simulink model "model_fully_coupled"  (R2021a)
settings: Solver=ode4  StartTime=0.0  StopTime=4  FixedStep=1e-2  RelTol=1e-3
values from neighbouring files (symbols this model uses):
  C_1 = [0.7887 -0.2113 -0.5774; -0.2113 0.7887 -0.5774; 0.5774 0.5774 0.5774]    [parameter.m]
  C_2 = [-0.2113 -0.5774 0.7887; 0.7887 -0.5774 -0.2113; 0.5774 0.5774 0.5774]    [parameter.m]
  C_3 = [-0.5774 0.7887 -0.2113; -0.5774 -0.2113 0.7887; 0.5774 0.5774 0.5774]    [parameter.m]
  d_1 = d    (= 4e-07)    [parameter.m]
  d_2 = d    (= 4e-07)    [parameter.m]
  d_3 = d    (= 4e-07)    [parameter.m]
  F = [0;0;0]    [parameter.m]
  g_s_1 = C_1(1:3,1)    [parameter.m]
  g_s_2 = C_2(1:3,1)    [parameter.m]
  g_s_3 = C_3(1:3,1)    [parameter.m]
  I = [1 0 0;0 1 0;0 0 1]    [parameter.m]
  I_hub_Bc = [550 0.1045 -0.0840; 0.1045 650 0.0001; -0.0840 0.0001 650]    [parameter.m]
  I_rw1_Wc1 = [1.5915E-4 0 1.54E-10; 0 0.8594E-4 0; 1.54E-10 0 0.8594E-4]    [parameter.m]
  I_rw1_Wc1_ = [0 -J_13_1 J_12_1; -J_13_1 (-2*J_23_1) (J_22_1-J_33_1); J_12_1 (J_22_1-J_33_1) (-2*J_23_1)]    [parameter.m]
  I_rw2_Wc2 = [1.5915E-4 0 1.54E-10; 0 0.8594E-4 0; 1.54E-10 0 0.8594E-4]    [parameter.m]
  I_rw2_Wc2_ = [0 -J_13_2 J_12_2; -J_13_2 (-2*J_23_2) (J_22_2-J_33_2); J_12_2 (J_22_2-J_33_2) (-2*J_23_2)]    [parameter.m]
  I_rw3_Wc3 = [1.5915E-4 0 1.54E-10; 0 0.8594E-4 0; 1.54E-10 0 0.8594E-4]    [parameter.m]
  I_rw3_Wc3_ = [0 -J_13_3 J_12_3; -J_13_3 (-2*J_23_3) (J_22_3-J_33_3); J_12_3 (J_22_3-J_33_3) (-2*J_23_3)]    [parameter.m]
  J_11_1 = I_rw1_Wc1(1,1)    [parameter.m]
  J_11_2 = I_rw2_Wc2(1,1)    [parameter.m]
  J_11_3 = I_rw3_Wc3(1,1)    [parameter.m]
  J_12_1 = I_rw1_Wc1(1,2)    [parameter.m]
  J_12_2 = I_rw2_Wc2(1,2)    [parameter.m]
  J_12_3 = I_rw3_Wc3(1,2)    [parameter.m]
  J_13_1 = I_rw1_Wc1(1,3)    [parameter.m]
  J_13_2 = I_rw2_Wc2(1,3)    [parameter.m]
  J_13_3 = I_rw3_Wc3(1,3)    [parameter.m]
  J_22_1 = I_rw1_Wc1(2,2)    [parameter.m]
  J_22_2 = I_rw2_Wc2(2,2)    [parameter.m]
  J_22_3 = I_rw3_Wc3(2,2)    [parameter.m]
  J_23_1 = I_rw1_Wc1(2,3)    [parameter.m]
  J_23_2 = I_rw2_Wc2(2,3)    [parameter.m]
  J_23_3 = I_rw3_Wc3(2,3)    [parameter.m]
  J_33_1 = I_rw1_Wc1(3,3)    [parameter.m]
  J_33_2 = I_rw2_Wc2(3,3)    [parameter.m]
  J_33_3 = I_rw3_Wc3(3,3)    [parameter.m]
  m_hub = 644    [parameter.m]
  m_rw_1 = m_rw(1)    [parameter.m]
  m_rw_2 = m_rw(2)    [parameter.m]
  m_rw_3 = m_rw(3)    [parameter.m]
  m_sc = 680    [parameter.m]
  OMEGA_1 = OMEGA(1)    [parameter.m]
  OMEGA_2 = OMEGA(2)    [parameter.m]
  OMEGA_3 = OMEGA(3)    [parameter.m]
  omega_BN = [omega ; omega; omega]    [parameter.m]
  r_Bc_B = [1e-2; -2e-2; 10e-2]    [parameter.m]
  r_BN = [0;0;0]    [parameter.m]
  r_W1_B = [0.6309; -0.1691; 0.4619]    [parameter.m]
  r_W2_B = [-0.1691; 0.6309; 0.4619]    [parameter.m]
  r_W3_B = [-0.4619; -0.4619; 0.4619]    [parameter.m]
  sigma_BN = [sigma; sigma; sigma]    [parameter.m]
  u_s_1 = u_s(1)    [parameter.m]
  u_s_2 = u_s(2)    [parameter.m]
  u_s_3 = u_s(3)    [parameter.m]
  w_2_1 = C_1(1:3,2)    [parameter.m]
  w_2_2 = C_2(1:3,2)    [parameter.m]
  w_2_3 = C_3(1:3,2)    [parameter.m]
  w_3_1 = C_1(1:3,3)    [parameter.m]
  w_3_2 = C_2(1:3,3)    [parameter.m]
  w_3_3 = C_3(1:3,3)    [parameter.m]
undefined symbols (not defined in the file or in its folder): deg, magnitude, rad, s
libraries: aerolibconvert2 x4, sharedutil x1, aerolibutil x1
(part 2 of 3)

== system model_fully_coupled/omega_dot_BN/6/1 ==
  I_rw1_Wc1 : Inport
  g_s_1 : Inport  Port=2
  m_rw_1 : Inport  Port=3
  OMEGA_1 : Inport  Port=4
  Add : Sum
  Matrix Multiply4 : Product  Multiplication=Matrix(*)
  Matrix Multiply5 : Product  Multiplication=Matrix(*)
  Product1 : Product
  Product2 : Product
  Out1 : Outport
  wires:
  Matrix Multiply4/1 -> Add/1
  Matrix Multiply5/1 -> Product2/2
  Product1/1 -> Matrix Multiply4/2
  Product2/1 -> Add/2
  g_s_1/1 -> Product1/2
  m_rw_1/1 -> Product2/1
  I_rw1_Wc1/1 -> Matrix Multiply4/1
  OMEGA_1/1 -> Product1/1
  Add/1 -> Out1/1
  [r_Wc1_B_skew] -> Matrix Multiply5/1
  [r_prime_Wc1_B] -> Matrix Multiply5/2

== system model_fully_coupled/omega_dot_BN/6/2 ==
  I_rw2_Wc2 : Inport
  g_s_2 : Inport  Port=2
  m_rw_2 : Inport  Port=3
  OMEGA_2 : Inport  Port=4
  Add1 : Sum
  Matrix Multiply1 : Product  Multiplication=Matrix(*)
  Matrix Multiply2 : Product  Multiplication=Matrix(*)
  Product3 : Product
  Product4 : Product
  Out2 : Outport
  wires:
  Matrix Multiply1/1 -> Add1/1
  Matrix Multiply2/1 -> Product4/2
  Product3/1 -> Matrix Multiply1/2
  I_rw2_Wc2/1 -> Matrix Multiply1/1
  m_rw_2/1 -> Product4/1
  Product4/1 -> Add1/2
  g_s_2/1 -> Product3/2
  Add1/1 -> Out2/1
  OMEGA_2/1 -> Product3/1
  [r_Wc2_B_skew] -> Matrix Multiply2/1
  [r_prime_Wc2_B] -> Matrix Multiply2/2

== system model_fully_coupled/omega_dot_BN/6/3 ==
  I_rw3_Wc3 : Inport
  g_s_3 : Inport  Port=2
  m_rw_3 : Inport  Port=3
  OMEGA_3 : Inport  Port=4
  Add2 : Sum
  Matrix Multiply3 : Product  Multiplication=Matrix(*)
  Matrix Multiply6 : Product  Multiplication=Matrix(*)
  Product5 : Product
  Product6 : Product
  Out3 : Outport
  wires:
  OMEGA_3/1 -> Product5/1
  Matrix Multiply3/1 -> Add2/1
  Matrix Multiply6/1 -> Product6/2
  m_rw_3/1 -> Product6/1
  Product6/1 -> Add2/2
  [r_Wc3_B_skew] -> Matrix Multiply6/1
  g_s_3/1 -> Product5/2
  I_rw3_Wc3/1 -> Matrix Multiply3/1
  Add2/1 -> Out3/1
  Product5/1 -> Matrix Multiply3/2
  [r_prime_Wc3_B] -> Matrix Multiply6/2

== system model_fully_coupled/omega_dot_BN/6/I_rwi_Wci ==
  Out1 : Outport
  Out2 : Outport  Port=2
  Out3 : Outport  Port=3
  wires:
  [I_rw1_Wc1] -> Out1/1
  [I_rw3_Wc3] -> Out3/1
  [I_rw2_Wc2] -> Out2/1

== system model_fully_coupled/omega_dot_BN/6/g_s_i ==
  g_s_1 : Constant  Value=g_s_1
  g_s_2 : Constant  Value=g_s_2
  g_s_3 : Constant  Value=g_s_3
  Out1 : Outport
  Out2 : Outport  Port=2
  Out3 : Outport  Port=3
  wires:
  g_s_3/1 -> Out3/1
  g_s_1/1 -> Out1/1
  g_s_2/1 -> Out2/1

== system model_fully_coupled/omega_dot_BN/6/m_rw_i ==
  m_rw_1 : Constant  Value=m_rw_1
  m_rw_2 : Constant  Value=m_rw_2
  m_rw_3 : Constant  Value=m_rw_3
  Out1 : Outport
  Out2 : Outport  Port=2
  Out3 : Outport  Port=3
  wires:
  m_rw_1/1 -> Out1/1
  m_rw_3/1 -> Out3/1
  m_rw_2/1 -> Out2/1

== system model_fully_coupled/omega_dot_BN/7 /m_rw_i ==
  m_rw_1 : Constant  Value=m_rw_1
  m_rw_2 : Constant  Value=m_rw_2
  m_rw_3 : Constant  Value=m_rw_3
  Out1 : Outport
  Out2 : Outport  Port=2
  Out3 : Outport  Port=3
  wires:
  m_rw_1/1 -> Out1/1
  m_rw_3/1 -> Out3/1
  m_rw_2/1 -> Out2/1

== system model_fully_coupled/r_double_dot_BN/c_double_dot/2 ==
  omega_BN : Inport
  c' : Inport  Port=2
  Gain : Gain  Gain=2
  Matrix Multiply1 : Product  Multiplication=Matrix(*)
  Subsystem1 : Subsystem
  1 : Outport
  tag scope: omega_BN_skew=global
  wires:
  omega_BN/1 -> Subsystem1/1(" ")
  Subsystem1/1("skew ") -> [omega_BN_skew], Matrix Multiply1/1
  c'/1 -> Matrix Multiply1/2
  Matrix Multiply1/1 -> Gain/1
  Gain/1 -> 1/1

== system model_fully_coupled/r_double_dot_BN/c_double_dot/3 ==
  omega_dot_BN : Inport
  c : Inport  Port=2
  Matrix Multiply1 : Product  Multiplication=Matrix(*)
  Subsystem1 : Subsystem
  1 : Outport
  wires:
  omega_dot_BN/1 -> Subsystem1/1(" ")
  Matrix Multiply1/1 -> 1/1
  Subsystem1/1("skew ") -> Matrix Multiply1/1
  c/1 -> Matrix Multiply1/2

== system model_fully_coupled/r_double_dot_BN/c_double_dot/4 ==
  c : Inport
  Matrix Multiply : Product  Multiplication=Matrix(*)
  Matrix Multiply1 : Product  Multiplication=Matrix(*)
  1 : Outport
  wires:
  Matrix Multiply/1 -> 1/1
  Matrix Multiply1/1 -> Matrix Multiply/2
  c/1 -> Matrix Multiply1/2
  [omega_BN_skew] -> Matrix Multiply1/1, Matrix Multiply/1

== system model_fully_coupled/r_double_dot_BN/c_double_dot/Subsystem1 ==
  In1 : Inport
  Demux : Demux  Outputs=3
  skew : MATLAB Function  TreatAsAtomicUnit=on
  "skew " : Outport
  wires:
  In1/1 -> Demux/1
  Demux/3 -> skew/3(a_3)
  Demux/2 -> skew/2(a_2)
  Demux/1 -> skew/1(a_1)
  skew/1(skew) -> "skew "/1

== system model_fully_coupled/r_double_dot_BN/c_double_dot/c ==
  Add : Sum  Inputs=+++
  Add1 : Sum
  Gain : Gain  Gain=1/m_sc
  Product{,1..3} (4 alike) : Product
  m_hub : Constant  Value=m_hub
  m_rw_i : Subsystem
  c : Outport
  wires:
  Add/1 -> Add1/2
  m_hub/1 -> Product/1
  Product1/1 -> Add/1
  [r_Bc_B] -> Product/2
  Product3/1 -> Add/3
  Product2/1 -> Add/2
  Product/1 -> Add1/1
  Add1/1 -> Gain/1
  Gain/1 -> c/1
  m_rw_i/1(Out1) -> Product1/1
  [r_Wc1_B] -> Product1/2
  m_rw_i/2(Out2) -> Product2/1
  [r_Wc2_B] -> Product2/2
  m_rw_i/3(Out3) -> Product3/1
  [r_Wc3_B] -> Product3/2

== system model_fully_coupled/r_double_dot_BN/c_double_dot/c" ==
  Add : Sum  Inputs=+++
  Gain : Gain  Gain=1/m_sc
  Product1 : Product
  Product2 : Product
  Product3 : Product
  m_rw_i : Subsystem
  "c\"" : Outport
  wires:
  Gain/1 -> "c\""/1
  Product1/1 -> Add/2
  Add/1 -> Gain/1
  Product2/1 -> Add/1
  Product3/1 -> Add/3
  [r_dprime_Wc1_B] -> Product2/2
  m_rw_i/1(Out1) -> Product2/1
  [r_dprime_Wc2_B] -> Product1/2
  m_rw_i/2(Out2) -> Product1/1
  m_rw_i/3(Out3) -> Product3/1
  [r_dprime_Wc3_B] -> Product3/2

== system model_fully_coupled/r_double_dot_BN/c_double_dot/c' ==
  Add : Sum  Inputs=+++
  Gain : Gain  Gain=1/m_sc
  Product1 : Product
  Product2 : Product
  Product3 : Product
  m_rw_i : Subsystem
  c' : Outport
  wires:
  Gain/1 -> c'/1
  Product1/1 -> Add/2
  Add/1 -> Gain/1
  Product2/1 -> Add/1
  Product3/1 -> Add/3
  [r_prime_Wc1_B] -> Product2/2
  m_rw_i/1(Out1) -> Product2/1
  [r_prime_Wc2_B] -> Product1/2
  m_rw_i/2(Out2) -> Product1/1
  m_rw_i/3(Out3) -> Product3/1
  [r_prime_Wc3_B] -> Product3/2

== system model_fully_coupled/r_double_dot_BN/c_double_dot/r_dprime_Wci_B ==
  OMEGA_1 : Inport
  OMEGA_2 : Inport  Port=2
  OMEGA_3 : Inport  Port=3
  w_2_1 : Inport  Port=4
  w_2_2 : Inport  Port=5
  w_2_3 : Inport  Port=6
  r_Wci_B' : Subsystem
  wires:
  w_2_3/1 -> r_Wci_B'/6(w_2_3)
  w_2_2/1 -> r_Wci_B'/5(w_2_2)
  w_2_1/1 -> r_Wci_B'/4(w_2_1)
  OMEGA_1/1 -> r_Wci_B'/1(OMEGA_1)
  OMEGA_2/1 -> r_Wci_B'/2(OMEGA_2)
  OMEGA_3/1 -> r_Wci_B'/3(OMEGA_3)

== system model_fully_coupled/r_double_dot_BN/c_double_dot/w_2_i dan w_3_i ==
  OMEGA_1 : Inport
  OMEGA_2 : Inport  Port=2
  OMEGA_3 : Inport  Port=3
  Subsystem : Subsystem
  Subsystem1 : Subsystem
  wires:
  OMEGA_1/1 -> Subsystem/1(OMEGA_1), Subsystem1/1(OMEGA_1)
  OMEGA_3/1 -> Subsystem/3(OMEGA_3), Subsystem1/3(OMEGA_3)
  OMEGA_2/1 -> Subsystem/2(OMEGA_2), Subsystem1/2(OMEGA_2)

== system model_fully_coupled/H_sc_B/2/H_rw1_B/Subsystem ==
  OMEGA_1 : Inport
  d_1 : Inport  Port=2
  w_3_1 : Inport  Port=3
  Add : Sum
  Matrix Multiply : Product  Multiplication=Matrix(*)
  Product1 : Product
  Product2 : Product
  Out1 : Outport
  wires:
  d_1/1 -> Product1/1
  Product1/1 -> Product2/2
  w_3_1/1 -> Product1/2
  [omega_BN_skew] -> Matrix Multiply/1
  OMEGA_1/1 -> Product2/1
  Product2/1 -> Add/1
  Matrix Multiply/1 -> Add/2
  Add/1 -> Out1/1
  [r_Wc1_B] -> Matrix Multiply/2

== system model_fully_coupled/H_sc_B/2/H_rw2_B/Subsystem ==
  OMEGA_2 : Inport
  d_2 : Inport  Port=2
  w_3_2 : Inport  Port=3
  Add : Sum
  Matrix Multiply : Product  Multiplication=Matrix(*)
  Product1 : Product
  Product2 : Product
  Out1 : Outport
  wires:
  d_2/1 -> Product1/1
  Product1/1 -> Product2/2
  w_3_2/1 -> Product1/2
  [omega_BN_skew] -> Matrix Multiply/1
  OMEGA_2/1 -> Product2/1
  Product2/1 -> Add/1
  Matrix Multiply/1 -> Add/2
  Add/1 -> Out1/1
  [r_Wc2_B] -> Matrix Multiply/2

== system model_fully_coupled/H_sc_B/2/H_rw3_B/Subsystem ==
  OMEGA_3 : Inport
  d_3 : Inport  Port=2
  w_3_3 : Inport  Port=3
  Add : Sum
  Matrix Multiply : Product  Multiplication=Matrix(*)
  Product1 : Product
  Product2 : Product
  Out1 : Outport
  wires:
  d_3/1 -> Product1/1
  Product1/1 -> Product2/2
  w_3_3/1 -> Product1/2
  [omega_BN_skew] -> Matrix Multiply/1
  OMEGA_3/1 -> Product2/1
  Product2/1 -> Add/1
  Matrix Multiply/1 -> Add/2
  Add/1 -> Out1/1
  [r_Wc3_B] -> Matrix Multiply/2

== system model_fully_coupled/OMEGA_dot_i/1/2/1 ==
  J_11_1 : Inport
  m_rw_1 : Inport  Port=2
  d_1 : Inport  Port=3
  g_s(T)_1 : Inport  Port=4
  Add : Sum
  Product : Product
  Product1 : Product
  Product3 : Product
  Out1 : Outport
  wires:
  g_s(T)_1/1 -> Product3/2
  m_rw_1/1 -> Product1/1
  Add/1 -> Product3/1
  Product/1 -> Product1/2
  Product1/1 -> Add/2
  Product3/1 -> Out1/1
  d_1/1 -> Product/2, Product/1
  J_11_1/1 -> Add/1

== system model_fully_coupled/OMEGA_dot_i/1/2/2 ==
  J_12_1 : Inport
  w_2(T)_1 : Inport  Port=2
  Product2 : Product
  Out1 : Outport
  wires:
  Product2/1 -> Out1/1
  J_12_1/1 -> Product2/1
  w_2(T)_1/1 -> Product2/2

== system model_fully_coupled/OMEGA_dot_i/1/2/3 ==
  J_13_1 : Inport
  w_3(T)_1 : Inport  Port=2
  Product2 : Product
  Out1 : Outport
  wires:
  Product2/1 -> Out1/1
  J_13_1/1 -> Product2/1
  w_3(T)_1/1 -> Product2/2

== system model_fully_coupled/OMEGA_dot_i/1/2/4 ==
  m_rw_1 : Inport
  d_1 : Inport  Port=2
  w_3(T)_1 : Inport  Port=3
  r_W1_B : Inport  Port=4
  omega_dot_BN : Inport  Port=5
  Matrix Multiply1 : Product  Multiplication=Matrix(*)
  Matrix Multiply2 : Product  Multiplication=Matrix(*)
  Product1 : Product
  Product3 : Product
  Subsystem1 : Subsystem
  Out1 : Outport
  wires:
  d_1/1 -> Product1/1
  Product1/1 -> Product3/2
  m_rw_1/1 -> Product3/1
  Product3/1 -> Out1/1
  r_W1_B/1 -> Subsystem1/1(r_W1_B)
  w_3(T)_1/1 -> Matrix Multiply2/1
  Subsystem1/1("skew ") -> Matrix Multiply2/2
  omega_dot_BN/1 -> Matrix Multiply1/2
  Matrix Multiply2/1 -> Matrix Multiply1/1
  Matrix Multiply1/1 -> Product1/2

== system model_fully_coupled/OMEGA_dot_i/1/Subsystem/w_s_1 ==
  omega_BN : Inport
  omega_dot_BN : Inport  Port=2
  g_s(T)_1 : Inport  Port=3
  Integrator : Integrator  InitialConditionSource=external
  Matrix Multiply1 : Product  Multiplication=Matrix(*)
  w_s_1 : Subsystem
  1 : Outport
  wires:
  g_s(T)_1/1 -> w_s_1/1(g_s(T)_1), Matrix Multiply1/1
  omega_dot_BN/1 -> Matrix Multiply1/2
  Matrix Multiply1/1 -> Integrator/1
  Integrator/1 -> 1/1
  omega_BN/1 -> w_s_1/2(omega_BN)
  w_s_1/1(Out1) -> Integrator/2

== system model_fully_coupled/OMEGA_dot_i/1/Subsystem/w_w_2_1 ==
  omega_BN : Inport
  omega_dot_BN : Inport  Port=2
  OMEGA_1 : Inport  Port=3
  w_2(T)_1 : Inport  Port=4
  Add : Sum
  Integrator : Integrator  InitialConditionSource=external
  Matrix Multiply1 : Product  Multiplication=Matrix(*)
  Product : Product
  w_w_2_1 : Subsystem
  1 : Outport
  tag scope: w_w_2_1=global
  wires:
  omega_BN/1 -> w_w_2_1/2(omega_BN)
  omega_dot_BN/1 -> Matrix Multiply1/2
  w_2(T)_1/1 -> w_w_2_1/1(w_2(T)_1), Matrix Multiply1/1
  w_w_2_1/1(Out1) -> Integrator/2
  Integrator/1 -> [w_w_2_1], 1/1
  OMEGA_1/1 -> Product/1
  Matrix Multiply1/1 -> Add/1
  Product/1 -> Add/2
  Add/1 -> Integrator/1
  [w_w_3_1] -> Product/2

== system model_fully_coupled/OMEGA_dot_i/1/Subsystem/w_w_3_1 ==
  omega_BN : Inport
  omega_dot_BN : Inport  Port=2
  OMEGA_1 : Inport  Port=3
  w_3(T)_1 : Inport  Port=4
  Add : Sum  Inputs=+-
  Integrator : Integrator  InitialConditionSource=external
  Matrix Multiply1 : Product  Multiplication=Matrix(*)
  Product : Product
  w_w_3_1 : Subsystem
  1 : Outport
  tag scope: w_w_3_1=global
  wires:
  w_w_3_1/1(Out1) -> Integrator/2
  Integrator/1 -> [w_w_3_1], 1/1
  Add/1 -> Integrator/1
  w_3(T)_1/1 -> w_w_3_1/1(w_3(T)_1), Matrix Multiply1/1
  omega_dot_BN/1 -> Matrix Multiply1/2
  OMEGA_1/1 -> Product/1
  omega_BN/1 -> w_w_3_1/2(omega_BN)
  Matrix Multiply1/1 -> Add/1
  Product/1 -> Add/2
  [w_w_2_1] -> Product/2

== system model_fully_coupled/OMEGA_dot_i/2/2/1 ==
  J_11_2 : Inport
  m_rw_2 : Inport  Port=2
  d_2 : Inport  Port=3
  g_s(T)_2 : Inport  Port=4
  Add : Sum
  Product : Product
  Product1 : Product
  Product3 : Product
  Out1 : Outport
  wires:
  g_s(T)_2/1 -> Product3/2
  m_rw_2/1 -> Product1/1
  Add/1 -> Product3/1
  Product/1 -> Product1/2
  Product1/1 -> Add/2
  Product3/1 -> Out1/1
  d_2/1 -> Product/2, Product/1
  J_11_2/1 -> Add/1

== system model_fully_coupled/OMEGA_dot_i/2/2/2 ==
  J_12_2 : Inport
  w_2(T)_2 : Inport  Port=2
  Product2 : Product
  Out1 : Outport
  wires:
  Product2/1 -> Out1/1
  J_12_2/1 -> Product2/1
  w_2(T)_2/1 -> Product2/2

== system model_fully_coupled/OMEGA_dot_i/2/2/3 ==
  J_13_2 : Inport
  w_3(T)_2 : Inport  Port=2
  Product2 : Product
  Out1 : Outport
  wires:
  Product2/1 -> Out1/1
  J_13_2/1 -> Product2/1
  w_3(T)_2/1 -> Product2/2

== system model_fully_coupled/OMEGA_dot_i/2/2/4 ==
  m_rw_2 : Inport
  d_2 : Inport  Port=2
  w_3(T)_2 : Inport  Port=3
  r_W2_B : Inport  Port=4
  omega_dot_BN : Inport  Port=5
  Matrix Multiply1 : Product  Multiplication=Matrix(*)
  Matrix Multiply2 : Product  Multiplication=Matrix(*)
  Product1 : Product
  Product3 : Product
  Subsystem1 : Subsystem
  Out1 : Outport
  wires:
  d_2/1 -> Product1/1
  Product1/1 -> Product3/2
  m_rw_2/1 -> Product3/1
  Product3/1 -> Out1/1
  r_W2_B/1 -> Subsystem1/1(r_W2_B)
  w_3(T)_2/1 -> Matrix Multiply2/1
  Subsystem1/1("skew ") -> Matrix Multiply2/2
  Matrix Multiply2/1 -> Matrix Multiply1/1
  omega_dot_BN/1 -> Matrix Multiply1/2
  Matrix Multiply1/1 -> Product1/2

== system model_fully_coupled/OMEGA_dot_i/2/Subsystem/w_s_2 ==
  omega_BN : Inport
  omega_dot_BN : Inport  Port=2
  g_s(T)_2 : Inport  Port=3
  Integrator : Integrator  InitialConditionSource=external
  Matrix Multiply1 : Product  Multiplication=Matrix(*)
  w_s_2 : Subsystem
  1 : Outport
  wires:
  g_s(T)_2/1 -> w_s_2/1(g_s(T)_2), Matrix Multiply1/1
  omega_dot_BN/1 -> Matrix Multiply1/2
  Matrix Multiply1/1 -> Integrator/1
  Integrator/1 -> 1/1
  omega_BN/1 -> w_s_2/2(omega_BN)
  w_s_2/1(Out1) -> Integrator/2

== system model_fully_coupled/OMEGA_dot_i/2/Subsystem/w_w_2_2 ==
  omega_BN : Inport
  omega_dot_BN : Inport  Port=2
  OMEGA_2 : Inport  Port=3
  w_2(T)_2 : Inport  Port=4
  Add : Sum
  Integrator : Integrator  InitialConditionSource=external
  Matrix Multiply1 : Product  Multiplication=Matrix(*)
  Product : Product
  w_w_2_2 : Subsystem
  1 : Outport
  tag scope: w_w_2_2=global
  wires:
  omega_BN/1 -> w_w_2_2/2(omega_BN)
  omega_dot_BN/1 -> Matrix Multiply1/2
  w_2(T)_2/1 -> w_w_2_2/1(w_2(T)_2), Matrix Multiply1/1
  w_w_2_2/1(Out1) -> Integrator/2
  Integrator/1 -> [w_w_2_2], 1/1
  OMEGA_2/1 -> Product/1
  Matrix Multiply1/1 -> Add/1
  Product/1 -> Add/2
  Add/1 -> Integrator/1
  [w_w_3_2] -> Product/2

== system model_fully_coupled/OMEGA_dot_i/2/Subsystem/w_w_3_2 ==
  omega_BN : Inport
  omega_dot_BN : Inport  Port=2
  OMEGA_2 : Inport  Port=3
  w_3(T)_2 : Inport  Port=4
  Add : Sum  Inputs=+-
  Integrator : Integrator  InitialConditionSource=external
  Matrix Multiply1 : Product  Multiplication=Matrix(*)
  Product : Product
  w_w_3_2 : Subsystem
  1 : Outport
  tag scope: w_w_3_2=global
  wires:
  w_w_3_2/1(Out1) -> Integrator/2
  Integrator/1 -> [w_w_3_2], 1/1
  Add/1 -> Integrator/1
  w_3(T)_2/1 -> w_w_3_2/1(w_3(T)_2), Matrix Multiply1/1
  omega_dot_BN/1 -> Matrix Multiply1/2
  OMEGA_2/1 -> Product/1
  omega_BN/1 -> w_w_3_2/2(omega_BN)
  Matrix Multiply1/1 -> Add/1
  Product/1 -> Add/2
  [w_w_2_2] -> Product/2

== system model_fully_coupled/OMEGA_dot_i/3/2/1 ==
  J_11_3 : Inport
  m_rw_3 : Inport  Port=2
  d_3 : Inport  Port=3
  g_s(T)_3 : Inport  Port=4
  Add : Sum
  Product : Product
  Product1 : Product
  Product3 : Product
  Out1 : Outport
  wires:
  g_s(T)_3/1 -> Product3/2
  m_rw_3/1 -> Product1/1
  Add/1 -> Product3/1
  Product/1 -> Product1/2
  Product1/1 -> Add/2
  Product3/1 -> Out1/1
  d_3/1 -> Product/2, Product/1
  J_11_3/1 -> Add/1

== system model_fully_coupled/OMEGA_dot_i/3/2/2 ==
  J_12_3 : Inport
  w_2(T)_3 : Inport  Port=2
  Product2 : Product
  Out1 : Outport
  wires:
  Product2/1 -> Out1/1
  J_12_3/1 -> Product2/1
  w_2(T)_3/1 -> Product2/2

== system model_fully_coupled/OMEGA_dot_i/3/2/3 ==
  J_13_3 : Inport
  w_3(T)_3 : Inport  Port=2
  Product2 : Product
  Out1 : Outport
  wires:
  Product2/1 -> Out1/1
  J_13_3/1 -> Product2/1
  w_3(T)_3/1 -> Product2/2

== system model_fully_coupled/OMEGA_dot_i/3/2/4 ==
  m_rw_3 : Inport
  d_3 : Inport  Port=2
  w_3(T)_3 : Inport  Port=3
  r_W3_B : Inport  Port=4
  omega_dot_BN : Inport  Port=5
  Matrix Multiply1 : Product  Multiplication=Matrix(*)
  Matrix Multiply2 : Product  Multiplication=Matrix(*)
  Product1 : Product
  Product3 : Product
  Subsystem1 : Subsystem
  Out1 : Outport
  wires:
  w_3(T)_3/1 -> Matrix Multiply2/1
  d_3/1 -> Product1/1
  Product1/1 -> Product3/2
  m_rw_3/1 -> Product3/1
  Product3/1 -> Out1/1
  r_W3_B/1 -> Subsystem1/1(r_W3_B)
  Subsystem1/1("skew ") -> Matrix Multiply2/2
  Matrix Multiply2/1 -> Matrix Multiply1/1
  omega_dot_BN/1 -> Matrix Multiply1/2
  Matrix Multiply1/1 -> Product1/2

== system model_fully_coupled/OMEGA_dot_i/3/Subsystem/w_s_3 ==
  omega_BN : Inport
  omega_dot_BN : Inport  Port=2
  g_s(T)_3 : Inport  Port=3
  Integrator : Integrator  InitialConditionSource=external
  Matrix Multiply1 : Product  Multiplication=Matrix(*)
  w_s_3 : Subsystem
  1 : Outport
  wires:
  g_s(T)_3/1 -> w_s_3/1(g_s(T)_3), Matrix Multiply1/1
  omega_dot_BN/1 -> Matrix Multiply1/2
  Matrix Multiply1/1 -> Integrator/1
  Integrator/1 -> 1/1
  omega_BN/1 -> w_s_3/2(omega_BN)
  w_s_3/1(Out1) -> Integrator/2

== system model_fully_coupled/OMEGA_dot_i/3/Subsystem/w_w_2_3 ==
  omega_BN : Inport
  omega_dot_BN : Inport  Port=2
  OMEGA_3 : Inport  Port=3
  w_2(T)_3 : Inport  Port=4
  Add : Sum
  Integrator : Integrator  InitialConditionSource=external
  Matrix Multiply1 : Product  Multiplication=Matrix(*)
  Product : Product
  w_w_2_3 : Subsystem
  1 : Outport
  tag scope: w_w_2_3=global
  wires:
  omega_BN/1 -> w_w_2_3/2(omega_BN)
  omega_dot_BN/1 -> Matrix Multiply1/2
  w_2(T)_3/1 -> w_w_2_3/1(w_2(T)_3), Matrix Multiply1/1
  w_w_2_3/1(Out1) -> Integrator/2
  Integrator/1 -> [w_w_2_3], 1/1
  OMEGA_3/1 -> Product/1
  Matrix Multiply1/1 -> Add/1
  Product/1 -> Add/2
  Add/1 -> Integrator/1
  [w_w_3_3] -> Product/2

== system model_fully_coupled/OMEGA_dot_i/3/Subsystem/w_w_3_3 ==
  omega_BN : Inport
  omega_dot_BN : Inport  Port=2
  OMEGA_3 : Inport  Port=3
  w_3(T)_3 : Inport  Port=4
  Add : Sum  Inputs=+-
  Integrator : Integrator  InitialConditionSource=external
  Matrix Multiply1 : Product  Multiplication=Matrix(*)
  Product : Product
  w_w_3_3 : Subsystem
  1 : Outport
  tag scope: w_w_3_3=global
  wires:
  w_w_3_3/1(Out1) -> Integrator/2
  Integrator/1 -> [w_w_3_3], 1/1
  Add/1 -> Integrator/1
  w_3(T)_3/1 -> w_w_3_3/1(w_3(T)_3), Matrix Multiply1/1
  omega_dot_BN/1 -> Matrix Multiply1/2
  OMEGA_3/1 -> Product/1
  omega_BN/1 -> w_w_3_3/2(omega_BN)
  Matrix Multiply1/1 -> Add/1
  Product/1 -> Add/2
  [w_w_2_3] -> Product/2

== system model_fully_coupled/omega_dot_BN/3/I_sc_B/I_hub_B ==
  Add : Sum
  I_hub_Bc : Constant  Value=I_hub_Bc
  Matrix Multiply : Product  Multiplication=Matrix(*)
  Product : Product
  Transpose : Math  Operator=transpose  SaturateOnIntegerOverflow=on
  m_hub : Constant  Value=m_hub
  Out1 : Outport
  wires:
  I_hub_Bc/1 -> Add/1
  Add/1 -> Out1/1
  [r_Bc_B_skew] -> Transpose/1, Matrix Multiply/1
  m_hub/1 -> Product/1
  Product/1 -> Add/2
  Matrix Multiply/1 -> Product/2
  Transpose/1 -> Matrix Multiply/2

== system model_fully_coupled/omega_dot_BN/3/I_sc_B/I_rwi_B ==
  OMEGA_1 : Inport
  OMEGA_2 : Inport  Port=2
  OMEGA_3 : Inport  Port=3
  Add : Sum  Inputs=+++
  I_rw1_B : Subsystem
  I_rw2_B : Subsystem
  I_rw3_B : Subsystem
  I_rwi_Wci : Subsystem
  m_rw_i : Subsystem
  Out1 : Outport
  wires:
  I_rw2_B/1(Out2) -> Add/2
  I_rw1_B/1(Out1) -> Add/1
  I_rw3_B/1(Out3) -> Add/3
  Add/1 -> Out1/1
  I_rwi_Wci/1(I_rw1_Wc1) -> I_rw1_B/1(I_rw1_Wc1)
  I_rwi_Wci/2(I_rw2_Wc2) -> I_rw2_B/1(I_rw2_Wc2)
  m_rw_i/1(Out1) -> I_rw1_B/2(m_rw_1)
  m_rw_i/2(Out2) -> I_rw2_B/2(m_rw_2)
  m_rw_i/3(Out3) -> I_rw3_B/2(m_rw_3)
  I_rwi_Wci/3(I_rw3_Wc3) -> I_rw3_B/1(I_rw3_Wc3)
  OMEGA_1/1 -> I_rwi_Wci/1(OMEGA_1)
  OMEGA_2/1 -> I_rwi_Wci/2(OMEGA_2)
  OMEGA_3/1 -> I_rwi_Wci/3(OMEGA_3)

== system model_fully_coupled/omega_dot_BN/3/I_sc_B'/I_rw1_B' ==
  I_rw1_Wc1' : Inport
  m_rw_1 : Inport  Port=2
  Add : Sum  Inputs=+++
  Matrix Multiply : Product  Multiplication=Matrix(*)
  Matrix Multiply1 : Product  Multiplication=Matrix(*)
  Product : Product
  Product1 : Product
  Transpose : Math  Operator=transpose  SaturateOnIntegerOverflow=on
  Transpose1 : Math  Operator=transpose  SaturateOnIntegerOverflow=on
  Out1 : Outport
  wires:
  Transpose/1 -> Matrix Multiply/2
  Transpose1/1 -> Matrix Multiply1/2
  [r_Wc1_B_skew] -> Matrix Multiply1/1, Transpose/1
  Matrix Multiply/1 -> Product/2
  m_rw_1/1 -> Product/1, Product1/1
  Product/1 -> Add/2
  [r_prime_Wc1_B_skew] -> Transpose1/1, Matrix Multiply/1
  Matrix Multiply1/1 -> Product1/2
  Product1/1 -> Add/3
  I_rw1_Wc1'/1 -> Add/1
  Add/1 -> Out1/1

== system model_fully_coupled/omega_dot_BN/3/I_sc_B'/I_rw2_B' ==
  I_rw2_Wc2' : Inport
  m_rw_2 : Inport  Port=2
  Add1 : Sum  Inputs=+++
  Matrix Multiply2 : Product  Multiplication=Matrix(*)
  Matrix Multiply3 : Product  Multiplication=Matrix(*)
  Product2 : Product
  Product3 : Product
  Transpose2 : Math  Operator=transpose  SaturateOnIntegerOverflow=on
  Transpose3 : Math  Operator=transpose  SaturateOnIntegerOverflow=on
  Out2 : Outport
  wires:
  Matrix Multiply3/1 -> Product3/2
  m_rw_2/1 -> Product3/1, Product2/1
  Product2/1 -> Add1/2
  Add1/1 -> Out2/1
  Transpose3/1 -> Matrix Multiply3/2
  [r_prime_Wc2_B_skew] -> Transpose3/1, Matrix Multiply2/1
  Transpose2/1 -> Matrix Multiply2/2
  [r_Wc2_B_skew] -> Matrix Multiply3/1, Transpose2/1
  I_rw2_Wc2'/1 -> Add1/1
  Product3/1 -> Add1/3
  Matrix Multiply2/1 -> Product2/2

== system model_fully_coupled/omega_dot_BN/3/I_sc_B'/I_rw3_B' ==
  I_rw3_Wc3' : Inport
  m_rw_3 : Inport  Port=2
  Add2 : Sum  Inputs=+++
  Matrix Multiply4 : Product  Multiplication=Matrix(*)
  Matrix Multiply5 : Product  Multiplication=Matrix(*)
  Product4 : Product
  Product5 : Product
  Transpose4 : Math  Operator=transpose  SaturateOnIntegerOverflow=on
  Transpose5 : Math  Operator=transpose  SaturateOnIntegerOverflow=on
  Out3 : Outport
  wires:
  Product5/1 -> Add2/3
  Add2/1 -> Out3/1
  Transpose5/1 -> Matrix Multiply5/2
  Transpose4/1 -> Matrix Multiply4/2
  m_rw_3/1 -> Product5/1, Product4/1
  Matrix Multiply5/1 -> Product5/2
  [r_Wc3_B_skew] -> Matrix Multiply5/1, Transpose4/1
  Matrix Multiply4/1 -> Product4/2
  I_rw3_Wc3'/1 -> Add2/1
  Product4/1 -> Add2/2
  [r_prime_Wc3_B_skew] -> Transpose5/1, Matrix Multiply4/1

== system model_fully_coupled/omega_dot_BN/3/I_sc_B'/I_rwi_Wci' ==
  1 : Outport
  2 : Outport  Port=2
  3 : Outport  Port=3
  wires:
  [I_rw1_Wc1_] -> 1/1
  [I_rw3_Wc3_] -> 3/1
  [I_rw2_Wc2_] -> 2/1

== system model_fully_coupled/omega_dot_BN/3/I_sc_B'/m_rw_i ==
  m_rw_1 : Constant  Value=m_rw_1
  m_rw_2 : Constant  Value=m_rw_2
  m_rw_3 : Constant  Value=m_rw_3
  Out1 : Outport
  Out2 : Outport  Port=2
  Out3 : Outport  Port=3
  wires:
  m_rw_1/1 -> Out1/1
  m_rw_3/1 -> Out3/1
  m_rw_2/1 -> Out2/1

== system model_fully_coupled/r_double_dot_BN/c_double_dot/2/Subsystem1 ==
  " " : Inport
  Demux : Demux  Outputs=3
  skew : MATLAB Function  TreatAsAtomicUnit=on
  "skew " : Outport
  wires:
  " "/1 -> Demux/1
  Demux/3 -> skew/3(a_3)
  Demux/2 -> skew/2(a_2)
  Demux/1 -> skew/1(a_1)
  skew/1(skew) -> "skew "/1

== system model_fully_coupled/r_double_dot_BN/c_double_dot/3/Subsystem1 ==
  " " : Inport
  Demux : Demux  Outputs=3
  skew : MATLAB Function  TreatAsAtomicUnit=on
  "skew " : Outport
  wires:
  " "/1 -> Demux/1
  Demux/3 -> skew/3(a_3)
  Demux/2 -> skew/2(a_2)
  Demux/1 -> skew/1(a_1)
  skew/1(skew) -> "skew "/1

== system model_fully_coupled/r_double_dot_BN/c_double_dot/c/m_rw_i ==
  m_rw_1 : Constant  Value=m_rw_1
  m_rw_2 : Constant  Value=m_rw_2
  m_rw_3 : Constant  Value=m_rw_3
  Out1 : Outport
  Out2 : Outport  Port=2
  Out3 : Outport  Port=3
  wires:
  m_rw_1/1 -> Out1/1
  m_rw_3/1 -> Out3/1
  m_rw_2/1 -> Out2/1

== system model_fully_coupled/r_double_dot_BN/c_double_dot/c"/m_rw_i ==
  m_rw_1 : Constant  Value=m_rw_1
  m_rw_2 : Constant  Value=m_rw_2
  m_rw_3 : Constant  Value=m_rw_3
  Out1 : Outport
  Out2 : Outport  Port=2
  Out3 : Outport  Port=3
  wires:
  m_rw_1/1 -> Out1/1
  m_rw_3/1 -> Out3/1
  m_rw_2/1 -> Out2/1

== system model_fully_coupled/r_double_dot_BN/c_double_dot/c'/m_rw_i ==
  m_rw_1 : Constant  Value=m_rw_1
  m_rw_2 : Constant  Value=m_rw_2
  m_rw_3 : Constant  Value=m_rw_3
  Out1 : Outport
  Out2 : Outport  Port=2
  Out3 : Outport  Port=3
  wires:
  m_rw_1/1 -> Out1/1
  m_rw_3/1 -> Out3/1
  m_rw_2/1 -> Out2/1

== system model_fully_coupled/r_double_dot_BN/c_double_dot/r_dprime_Wci_B/r_Wci_B' ==
  OMEGA_1 : Inport
  OMEGA_2 : Inport  Port=2
  OMEGA_3 : Inport  Port=3
  w_2_1 : Inport  Port=4
  w_2_2 : Inport  Port=5
  w_2_3 : Inport  Port=6
  Subsystem : Subsystem
  Subsystem1 : Subsystem
  Subsystem2 : Subsystem
  d_i : Subsystem
  g_s_i : Subsystem
  wires:
  d_i/1(Out1) -> Subsystem/1(d_1)
  d_i/2(Out2) -> Subsystem1/1(d_2)
  d_i/3(Out3) -> Subsystem2/1(d_3)
  w_2_1/1 -> Subsystem/2(w_2_1)
  w_2_2/1 -> Subsystem1/2(w_2_2)
  w_2_3/1 -> Subsystem2/2(w_2_3)
  OMEGA_1/1 -> Subsystem/3(OMEGA_1)
  OMEGA_2/1 -> Subsystem1/3(OMEGA_2)
  OMEGA_3/1 -> Subsystem2/3(OMEGA_3)
  g_s_i/1(Out1) -> Subsystem/4(g_s_1)
  g_s_i/2(Out2) -> Subsystem1/4(g_s_2)
  g_s_i/3(Out3) -> Subsystem2/4(g_s_3)

== system model_fully_coupled/r_double_dot_BN/c_double_dot/w_2_i dan w_3_i/Subsystem ==
  OMEGA_1 : Inport
  OMEGA_2 : Inport  Port=2
  OMEGA_3 : Inport  Port=3
  Constant3 : Constant  Value=w_3_1
  Constant4 : Constant  Value=w_3_2
  Constant5 : Constant  Value=w_3_3
  Integrator4 : Integrator  InitialConditionSource=external
  Integrator5 : Integrator  InitialConditionSource=external
  Integrator6 : Integrator  InitialConditionSource=external
  w_3_1' : Subsystem
  w_3_2' : Subsystem
  w_3_3' : Subsystem
  tag scope: w_3_1=global, w_3_2=global, w_3_3=global
  wires:
  Integrator4/1 -> [w_3_1]
  OMEGA_1/1 -> w_3_1'/1(OMEGA_1)
  Constant4/1 -> Integrator5/2
  w_3_1'/1(Out1) -> Integrator4/1
  Constant3/1 -> Integrator4/2
  w_3_3'/1(Out1) -> Integrator6/1
  Integrator5/1 -> [w_3_2]
  OMEGA_2/1 -> w_3_2'/1(OMEGA_2)
  Constant5/1 -> Integrator6/2
  w_3_2'/1(Out1) -> Integrator5/1
  OMEGA_3/1 -> w_3_3'/1(OMEGA_3)
  Integrator6/1 -> [w_3_3]
  [w_2_1] -> w_3_1'/2(w_2_1)
  [w_2_2] -> w_3_2'/2(w_2_2)
  [w_2_3] -> w_3_3'/2(w_2_3)

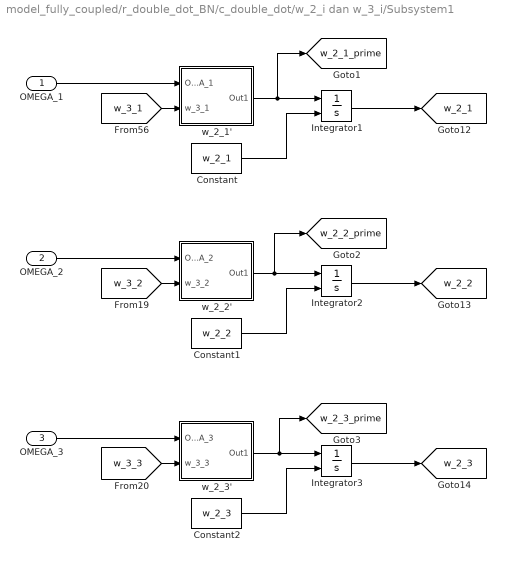
== system model_fully_coupled/r_double_dot_BN/c_double_dot/w_2_i dan w_3_i/Subsystem1 ==
  OMEGA_1 : Inport
  OMEGA_2 : Inport  Port=2
  OMEGA_3 : Inport  Port=3
  Constant : Constant  Value=w_2_1
  Constant1 : Constant  Value=w_2_2
  Constant2 : Constant  Value=w_2_3
  Integrator1 : Integrator  InitialConditionSource=external
  Integrator2 : Integrator  InitialConditionSource=external
  Integrator3 : Integrator  InitialConditionSource=external
  w_2_1' : Subsystem
  w_2_2' : Subsystem
  w_2_3' : Subsystem
  tag scope: w_2_1=global, w_2_1_prime=global, w_2_2=global, w_2_2_prime=global, w_2_3=global, w_2_3_prime=global
  wires:
  w_2_1'/1(Out1) -> [w_2_1_prime], Integrator1/1
  OMEGA_1/1 -> w_2_1'/1(OMEGA_1)
  Integrator1/1 -> [w_2_1]
  Constant/1 -> Integrator1/2
  Constant1/1 -> Integrator2/2
  Integrator2/1 -> [w_2_2]
  OMEGA_2/1 -> w_2_2'/1(OMEGA_2)
  w_2_2'/1(Out1) -> [w_2_2_prime], Integrator2/1
  Constant2/1 -> Integrator3/2
  Integrator3/1 -> [w_2_3]
  OMEGA_3/1 -> w_2_3'/1(OMEGA_3)
  w_2_3'/1(Out1) -> [w_2_3_prime], Integrator3/1
  [w_3_1] -> w_2_1'/2(w_3_1)
  [w_3_2] -> w_2_2'/2(w_3_2)
  [w_3_3] -> w_2_3'/2(w_3_3)

== system model_fully_coupled/OMEGA_dot_i/1/2/4/Subsystem1 ==
  r_W1_B : Inport
  Demux : Demux  Outputs=3
  skew : MATLAB Function  TreatAsAtomicUnit=on
  "skew " : Outport
  wires:
  r_W1_B/1 -> Demux/1
  Demux/3 -> skew/3(a_3)
  Demux/2 -> skew/2(a_2)
  Demux/1 -> skew/1(a_1)
  skew/1(skew) -> "skew "/1

== system model_fully_coupled/OMEGA_dot_i/1/Subsystem/w_s_1/w_s_1 ==
  g_s(T)_1 : Inport
  omega_BN : Inport  Port=2
  Matrix Multiply2 : Product  Multiplication=Matrix(*)
  Out1 : Outport
  wires:
  omega_BN/1 -> Matrix Multiply2/2
  g_s(T)_1/1 -> Matrix Multiply2/1
  Matrix Multiply2/1 -> Out1/1

== system model_fully_coupled/OMEGA_dot_i/1/Subsystem/w_w_2_1/w_w_2_1 ==
  w_2(T)_1 : Inport
  omega_BN : Inport  Port=2
  Matrix Multiply1 : Product  Multiplication=Matrix(*)
  Out1 : Outport
  wires:
  w_2(T)_1/1 -> Matrix Multiply1/1
  Matrix Multiply1/1 -> Out1/1
  omega_BN/1 -> Matrix Multiply1/2

== system model_fully_coupled/OMEGA_dot_i/1/Subsystem/w_w_3_1/w_w_3_1 ==
  w_3(T)_1 : Inport
  omega_BN : Inport  Port=2
  Matrix Multiply1 : Product  Multiplication=Matrix(*)
  Out1 : Outport
  wires:
  w_3(T)_1/1 -> Matrix Multiply1/1
  Matrix Multiply1/1 -> Out1/1
  omega_BN/1 -> Matrix Multiply1/2

== system model_fully_coupled/OMEGA_dot_i/2/2/4/Subsystem1 ==
  r_W2_B : Inport
  Demux : Demux  Outputs=3
  skew : MATLAB Function  TreatAsAtomicUnit=on
  "skew " : Outport
  wires:
  r_W2_B/1 -> Demux/1
  Demux/3 -> skew/3(a_3)
  Demux/2 -> skew/2(a_2)
  Demux/1 -> skew/1(a_1)
  skew/1(skew) -> "skew "/1

== system model_fully_coupled/OMEGA_dot_i/2/Subsystem/w_s_2/w_s_2 ==
  g_s(T)_2 : Inport
  omega_BN : Inport  Port=2
  Matrix Multiply2 : Product  Multiplication=Matrix(*)
  Out1 : Outport
  wires:
  omega_BN/1 -> Matrix Multiply2/2
  g_s(T)_2/1 -> Matrix Multiply2/1
  Matrix Multiply2/1 -> Out1/1

== system model_fully_coupled/OMEGA_dot_i/2/Subsystem/w_w_2_2/w_w_2_2 ==
  w_2(T)_2 : Inport
  omega_BN : Inport  Port=2
  Matrix Multiply1 : Product  Multiplication=Matrix(*)
  Out1 : Outport
  wires:
  w_2(T)_2/1 -> Matrix Multiply1/1
  Matrix Multiply1/1 -> Out1/1
  omega_BN/1 -> Matrix Multiply1/2

== system model_fully_coupled/OMEGA_dot_i/2/Subsystem/w_w_3_2/w_w_3_2 ==
  w_3(T)_2 : Inport
  omega_BN : Inport  Port=2
  Matrix Multiply1 : Product  Multiplication=Matrix(*)
  Out1 : Outport
  wires:
  w_3(T)_2/1 -> Matrix Multiply1/1
  Matrix Multiply1/1 -> Out1/1
  omega_BN/1 -> Matrix Multiply1/2

== system model_fully_coupled/OMEGA_dot_i/3/2/4/Subsystem1 ==
  r_W3_B : Inport
  Demux : Demux  Outputs=3
  skew : MATLAB Function  TreatAsAtomicUnit=on
  "skew " : Outport
  wires:
  r_W3_B/1 -> Demux/1
  Demux/3 -> skew/3(a_3)
  Demux/2 -> skew/2(a_2)
  Demux/1 -> skew/1(a_1)
  skew/1(skew) -> "skew "/1

== system model_fully_coupled/OMEGA_dot_i/3/Subsystem/w_s_3/w_s_3 ==
  g_s(T)_3 : Inport
  omega_BN : Inport  Port=2
  Matrix Multiply2 : Product  Multiplication=Matrix(*)
  Out1 : Outport
  wires:
  omega_BN/1 -> Matrix Multiply2/2
  g_s(T)_3/1 -> Matrix Multiply2/1
  Matrix Multiply2/1 -> Out1/1

== system model_fully_coupled/OMEGA_dot_i/3/Subsystem/w_w_2_3/w_w_2_3 ==
  w_2(T)_3 : Inport
  omega_BN : Inport  Port=2
  Matrix Multiply1 : Product  Multiplication=Matrix(*)
  Out1 : Outport
  wires:
  w_2(T)_3/1 -> Matrix Multiply1/1
  Matrix Multiply1/1 -> Out1/1
  omega_BN/1 -> Matrix Multiply1/2

== system model_fully_coupled/OMEGA_dot_i/3/Subsystem/w_w_3_3/w_w_3_3 ==
  w_3(T)_3 : Inport
  omega_BN : Inport  Port=2
  Matrix Multiply1 : Product  Multiplication=Matrix(*)
  Out1 : Outport
  wires:
  w_3(T)_3/1 -> Matrix Multiply1/1
  Matrix Multiply1/1 -> Out1/1
  omega_BN/1 -> Matrix Multiply1/2

== system model_fully_coupled/omega_dot_BN/3/I_sc_B/I_rwi_B/I_rw1_B ==
  I_rw1_Wc1 : Inport
  m_rw_1 : Inport  Port=2
  Add : Sum
  Matrix Multiply : Product  Multiplication=Matrix(*)
  Product : Product
  Transpose : Math  Operator=transpose  SaturateOnIntegerOverflow=on
  Out1 : Outport
  wires:
  I_rw1_Wc1/1 -> Add/1
  Transpose/1 -> Matrix Multiply/2
  Product/1 -> Add/2
  [r_Wc1_B_skew] -> Matrix Multiply/1, Transpose/1
  Matrix Multiply/1 -> Product/2
  m_rw_1/1 -> Product/1
  Add/1 -> Out1/1

== system model_fully_coupled/omega_dot_BN/3/I_sc_B/I_rwi_B/I_rw2_B ==
  I_rw2_Wc2 : Inport
  m_rw_2 : Inport  Port=2
  Add1 : Sum
  Matrix Multiply1 : Product  Multiplication=Matrix(*)
  Product1 : Product
  Transpose1 : Math  Operator=transpose  SaturateOnIntegerOverflow=on
  Out2 : Outport
  wires:
  m_rw_2/1 -> Product1/1
  Transpose1/1 -> Matrix Multiply1/2
  Matrix Multiply1/1 -> Product1/2
  I_rw2_Wc2/1 -> Add1/1
  Product1/1 -> Add1/2
  Add1/1 -> Out2/1
  [r_Wc2_B_skew] -> Matrix Multiply1/1, Transpose1/1

== system model_fully_coupled/omega_dot_BN/3/I_sc_B/I_rwi_B/I_rw3_B ==
  I_rw3_Wc3 : Inport
  m_rw_3 : Inport  Port=2
  Add2 : Sum
  Matrix Multiply2 : Product  Multiplication=Matrix(*)
  Product2 : Product
  Transpose2 : Math  Operator=transpose  SaturateOnIntegerOverflow=on
  Out3 : Outport
  wires:
  m_rw_3/1 -> Product2/1
  Transpose2/1 -> Matrix Multiply2/2
  Matrix Multiply2/1 -> Product2/2
  I_rw3_Wc3/1 -> Add2/1
  [r_Wc3_B_skew] -> Matrix Multiply2/1, Transpose2/1
  Product2/1 -> Add2/2
  Add2/1 -> Out3/1

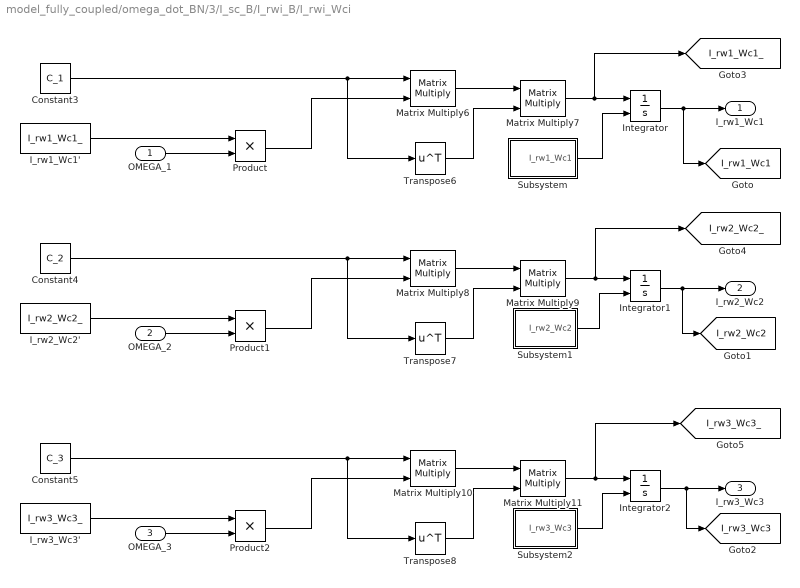
== system model_fully_coupled/omega_dot_BN/3/I_sc_B/I_rwi_B/I_rwi_Wci ==
  OMEGA_1 : Inport
  OMEGA_2 : Inport  Port=2
  OMEGA_3 : Inport  Port=3
  Constant3 : Constant  Value=C_1
  Constant4 : Constant  Value=C_2
  Constant5 : Constant  Value=C_3
  "I_rw1_Wc1' " : Constant  Value=I_rw1_Wc1_
  "I_rw2_Wc2' " : Constant  Value=I_rw2_Wc2_
  "I_rw3_Wc3' " : Constant  Value=I_rw3_Wc3_
  Integrator : Integrator  InitialConditionSource=external
  Integrator1 : Integrator  InitialConditionSource=external
  Integrator2 : Integrator  InitialConditionSource=external
  Matrix Multiply{6..11} (6 alike) : Product  Multiplication=Matrix(*)
  Product : Product
  Product1 : Product
  Product2 : Product
  Subsystem : Subsystem
  Subsystem1 : Subsystem
  Subsystem2 : Subsystem
  Transpose6 : Math  Operator=transpose  SaturateOnIntegerOverflow=on
  Transpose7 : Math  Operator=transpose  SaturateOnIntegerOverflow=on
  Transpose8 : Math  Operator=transpose  SaturateOnIntegerOverflow=on
  I_rw1_Wc1 : Outport
  I_rw2_Wc2 : Outport  Port=2
  I_rw3_Wc3 : Outport  Port=3
  tag scope: I_rw1_Wc1=global, I_rw1_Wc1_=global, I_rw2_Wc2=global, I_rw2_Wc2_=global, I_rw3_Wc3=global, I_rw3_Wc3_=global
  wires:
  OMEGA_3/1 -> Product2/2
  Product2/1 -> Matrix Multiply10/2
  Matrix Multiply10/1 -> Matrix Multiply11/1
  "I_rw1_Wc1' "/1 -> Product/1
  OMEGA_1/1 -> Product/2
  Matrix Multiply6/1 -> Matrix Multiply7/1
  Matrix Multiply7/1 -> Integrator/1, [I_rw1_Wc1_]
  Constant4/1 -> Transpose7/1, Matrix Multiply8/1
  Transpose7/1 -> Matrix Multiply9/2
  Product/1 -> Matrix Multiply6/2
  Constant3/1 -> Transpose6/1, Matrix Multiply6/1
  OMEGA_2/1 -> Product1/2
  "I_rw2_Wc2' "/1 -> Product1/1
  "I_rw3_Wc3' "/1 -> Product2/1
  Product1/1 -> Matrix Multiply8/2
  Matrix Multiply8/1 -> Matrix Multiply9/1
  Transpose8/1 -> Matrix Multiply11/2
  Matrix Multiply9/1 -> Integrator1/1, [I_rw2_Wc2_]
  Constant5/1 -> Transpose8/1, Matrix Multiply10/1
  Transpose6/1 -> Matrix Multiply7/2
  Matrix Multiply11/1 -> Integrator2/1, [I_rw3_Wc3_]
  Integrator/1 -> [I_rw1_Wc1], I_rw1_Wc1/1
  Subsystem/1(I_rw1_Wc1) -> Integrator/2
  Integrator1/1 -> [I_rw2_Wc2], I_rw2_Wc2/1
  Subsystem1/1(I_rw2_Wc2) -> Integrator1/2
  Integrator2/1 -> [I_rw3_Wc3], I_rw3_Wc3/1
  Subsystem2/1(I_rw3_Wc3) -> Integrator2/2

== system model_fully_coupled/omega_dot_BN/3/I_sc_B/I_rwi_B/m_rw_i ==
  m_rw_1 : Constant  Value=m_rw_1
  m_rw_2 : Constant  Value=m_rw_2
  m_rw_3 : Constant  Value=m_rw_3
  Out1 : Outport
  Out2 : Outport  Port=2
  Out3 : Outport  Port=3
  wires:
  m_rw_1/1 -> Out1/1
  m_rw_3/1 -> Out3/1
  m_rw_2/1 -> Out2/1

== system model_fully_coupled/r_double_dot_BN/c_double_dot/r_dprime_Wci_B/r_Wci_B'/Subsystem ==
  d_1 : Inport
  w_2_1 : Inport  Port=2
  OMEGA_1 : Inport  Port=3
  g_s_1 : Inport  Port=4
  Constant : Constant  Value=r_W1_B
  Integrator : Integrator  InitialConditionSource=external
  Integrator1 : Integrator  InitialConditionSource=external
  Subsystem1 : Subsystem
  Subsystem2 : Subsystem
  "r\"_Wc1_B" : Subsystem
  r'_Wc1_B : Subsystem
  r_Wc1_B : Subsystem
  tag scope: r_Wc1_B=global, r_Wc1_B_skew=global, r_prime_Wc1_B=global, r_prime_Wc1_B_skew=global
  wires:
  d_1/1 -> r_Wc1_B/2(d_1), r'_Wc1_B/1(d_1)
  Subsystem1/1("skew ") -> [r_prime_Wc1_B_skew]
  Subsystem2/1("skew ") -> [r_Wc1_B_skew]
  Integrator/1 -> [r_Wc1_B], Subsystem2/1(1)
  Constant/1 -> r_Wc1_B/1(r_W1_B)
  w_2_1/1 -> r_Wc1_B/3(w_2_1)
  r_Wc1_B/1(1) -> Integrator/2
  "r\"_Wc1_B"/1(Out1) -> Integrator1/1
  r'_Wc1_B/1(1) -> Integrator1/2
  Integrator1/1 -> Subsystem1/1(1), [r_prime_Wc1_B], Integrator/1
  OMEGA_1/1 -> "r\"_Wc1_B"/1(OMEGA_1)
  g_s_1/1 -> "r\"_Wc1_B"/2(g_s_1)

== system model_fully_coupled/r_double_dot_BN/c_double_dot/r_dprime_Wci_B/r_Wci_B'/Subsystem1 ==
  d_2 : Inport
  w_2_2 : Inport  Port=2
  OMEGA_2 : Inport  Port=3
  g_s_2 : Inport  Port=4
  Constant : Constant  Value=r_W2_B
  Integrator : Integrator  InitialConditionSource=external
  Integrator1 : Integrator  InitialConditionSource=external
  Subsystem1 : Subsystem
  Subsystem2 : Subsystem
  "r\"_Wc2_B" : Subsystem
  r'_Wc2_B : Subsystem
  r_Wc2_B : Subsystem
  tag scope: r_Wc2_B=global, r_Wc2_B_skew=global, r_prime_Wc2_B=global, r_prime_Wc2_B_skew=global
  wires:
  d_2/1 -> r_Wc2_B/2(d_2), r'_Wc2_B/1(d_2)
  Subsystem1/1("skew ") -> [r_prime_Wc2_B_skew]
  Subsystem2/1("skew ") -> [r_Wc2_B_skew]
  r_Wc2_B/1(1) -> Integrator/2
  Integrator/1 -> [r_Wc2_B], Subsystem2/1(1)
  Constant/1 -> r_Wc2_B/1(r_W2_B)
  w_2_2/1 -> r_Wc2_B/3(w_2_2)
  "r\"_Wc2_B"/1(Out1) -> Integrator1/1
  r'_Wc2_B/1(1) -> Integrator1/2
  Integrator1/1 -> Subsystem1/1(1), [r_prime_Wc2_B], Integrator/1
  OMEGA_2/1 -> "r\"_Wc2_B"/1(OMEGA_2)
  g_s_2/1 -> "r\"_Wc2_B"/2(g_s_2)

== system model_fully_coupled/r_double_dot_BN/c_double_dot/r_dprime_Wci_B/r_Wci_B'/Subsystem2 ==
  d_3 : Inport
  w_2_3 : Inport  Port=2
  OMEGA_3 : Inport  Port=3
  g_s_3 : Inport  Port=4
  Constant : Constant  Value=r_W3_B
  Integrator : Integrator  InitialConditionSource=external
  Integrator1 : Integrator  InitialConditionSource=external
  Subsystem1 : Subsystem
  Subsystem2 : Subsystem
  "r\"_Wc3_B" : Subsystem
  r'_Wc3_B : Subsystem
  r_Wc3_B : Subsystem
  tag scope: r_Wc3_B=global, r_Wc3_B_skew=global, r_prime_Wc3_B=global, r_prime_Wc3_B_skew=global
  wires:
  d_3/1 -> r_Wc3_B/2(d_3), r'_Wc3_B/1(d_3)
  r'_Wc3_B/1(1) -> Integrator1/2
  Subsystem1/1("skew ") -> [r_prime_Wc3_B_skew]
  Subsystem2/1("skew ") -> [r_Wc3_B_skew]
  Integrator/1 -> [r_Wc3_B], Subsystem2/1(1)
  r_Wc3_B/1(1) -> Integrator/2
  Constant/1 -> r_Wc3_B/1(r_W3_B)
  w_2_3/1 -> r_Wc3_B/3(w_2_3)
  "r\"_Wc3_B"/1(Out1) -> Integrator1/1
  Integrator1/1 -> [r_prime_Wc3_B], Subsystem1/1(1), Integrator/1
  OMEGA_3/1 -> "r\"_Wc3_B"/1(OMEGA_3)
  g_s_3/1 -> "r\"_Wc3_B"/2(g_s_3)

== system model_fully_coupled/r_double_dot_BN/c_double_dot/r_dprime_Wci_B/r_Wci_B'/d_i ==
  d_1 : Constant  Value=d_1
  d_2 : Constant  Value=d_2
  d_3 : Constant  Value=d_3
  Out1 : Outport
  Out2 : Outport  Port=2
  Out3 : Outport  Port=3
  wires:
  d_3/1 -> Out3/1
  d_1/1 -> Out1/1
  d_2/1 -> Out2/1

== system model_fully_coupled/r_double_dot_BN/c_double_dot/r_dprime_Wci_B/r_Wci_B'/g_s_i ==
  g_s_1 : Constant  Value=g_s_1
  g_s_2 : Constant  Value=g_s_2
  g_s_3 : Constant  Value=g_s_3
  Out1 : Outport
  Out2 : Outport  Port=2
  Out3 : Outport  Port=3
  wires:
  g_s_3/1 -> Out3/1
  g_s_1/1 -> Out1/1
  g_s_2/1 -> Out2/1

== system model_fully_coupled/r_double_dot_BN/c_double_dot/w_2_i dan w_3_i/Subsystem/w_3_1' ==
  OMEGA_1 : Inport
  w_2_1 : Inport  Port=2
  Gain : Gain  Gain=-1
  Product : Product
  Out1 : Outport
  wires:
  w_2_1/1 -> Product/2
  Product/1 -> Out1/1
  Gain/1 -> Product/1
  OMEGA_1/1 -> Gain/1

== system model_fully_coupled/r_double_dot_BN/c_double_dot/w_2_i dan w_3_i/Subsystem/w_3_2' ==
  OMEGA_2 : Inport
  w_2_2 : Inport  Port=2
  Gain : Gain  Gain=-1
  Product : Product
  Out1 : Outport
  wires:
  w_2_2/1 -> Product/2
  Product/1 -> Out1/1
  Gain/1 -> Product/1
  OMEGA_2/1 -> Gain/1

== system model_fully_coupled/r_double_dot_BN/c_double_dot/w_2_i dan w_3_i/Subsystem/w_3_3' ==
  OMEGA_3 : Inport
  w_2_3 : Inport  Port=2
  Gain : Gain  Gain=-1
  Product : Product
  Out1 : Outport
  wires:
  w_2_3/1 -> Product/2
  Product/1 -> Out1/1
  Gain/1 -> Product/1
  OMEGA_3/1 -> Gain/1

== system model_fully_coupled/r_double_dot_BN/c_double_dot/w_2_i dan w_3_i/Subsystem1/w_2_1' ==
  OMEGA_1 : Inport
  w_3_1 : Inport  Port=2
  Product : Product
  Out1 : Outport
  wires:
  w_3_1/1 -> Product/2
  OMEGA_1/1 -> Product/1
  Product/1 -> Out1/1

== system model_fully_coupled/r_double_dot_BN/c_double_dot/w_2_i dan w_3_i/Subsystem1/w_2_2' ==
  OMEGA_2 : Inport
  w_3_2 : Inport  Port=2
  Product : Product
  Out1 : Outport
  wires:
  w_3_2/1 -> Product/2
  OMEGA_2/1 -> Product/1
  Product/1 -> Out1/1

== system model_fully_coupled/r_double_dot_BN/c_double_dot/w_2_i dan w_3_i/Subsystem1/w_2_3' ==
  OMEGA_3 : Inport
  w_3_3 : Inport  Port=2
  Product : Product
  Out1 : Outport
  wires:
  w_3_3/1 -> Product/2
  OMEGA_3/1 -> Product/1
  Product/1 -> Out1/1

== system model_fully_coupled/omega_dot_BN/3/I_sc_B/I_rwi_B/I_rwi_Wci/Subsystem ==
  Constant : Constant  Value=C_1
  "I_rw1_Wc1 " : Constant  Value=I_rw1_Wc1
  Matrix Multiply : Product  Multiplication=Matrix(*)
  Matrix Multiply1 : Product  Multiplication=Matrix(*)
  Transpose : Math  Operator=transpose  SaturateOnIntegerOverflow=on
  I_rw1_Wc1 : Outport
  wires:
  Transpose/1 -> Matrix Multiply1/2
  Matrix Multiply/1 -> Matrix Multiply1/1
  "I_rw1_Wc1 "/1 -> Matrix Multiply/2
  Constant/1 -> Transpose/1, Matrix Multiply/1
  Matrix Multiply1/1 -> I_rw1_Wc1/1

== system model_fully_coupled/omega_dot_BN/3/I_sc_B/I_rwi_B/I_rwi_Wci/Subsystem1 ==
  Constant1 : Constant  Value=C_2
  "I_rw2_Wc2 " : Constant  Value=I_rw2_Wc2
  Matrix Multiply2 : Product  Multiplication=Matrix(*)
  Matrix Multiply3 : Product  Multiplication=Matrix(*)
  Transpose1 : Math  Operator=transpose  SaturateOnIntegerOverflow=on
  I_rw2_Wc2 : Outport
  wires:
  Matrix Multiply2/1 -> Matrix Multiply3/1
  Matrix Multiply3/1 -> I_rw2_Wc2/1
  Transpose1/1 -> Matrix Multiply3/2
  "I_rw2_Wc2 "/1 -> Matrix Multiply2/2
  Constant1/1 -> Transpose1/1, Matrix Multiply2/1

== system model_fully_coupled/omega_dot_BN/3/I_sc_B/I_rwi_B/I_rwi_Wci/Subsystem2 ==
  Constant2 : Constant  Value=C_3
  "I_rw3_Wc3 " : Constant  Value=I_rw3_Wc3
  Matrix Multiply4 : Product  Multiplication=Matrix(*)
  Matrix Multiply5 : Product  Multiplication=Matrix(*)
  Transpose2 : Math  Operator=transpose  SaturateOnIntegerOverflow=on
  I_rw3_Wc3 : Outport
  wires:
  "I_rw3_Wc3 "/1 -> Matrix Multiply4/2
  Matrix Multiply5/1 -> I_rw3_Wc3/1
  Transpose2/1 -> Matrix Multiply5/2
  Constant2/1 -> Transpose2/1, Matrix Multiply4/1
  Matrix Multiply4/1 -> Matrix Multiply5/1

== system model_fully_coupled/r_double_dot_BN/c_double_dot/r_dprime_Wci_B/r_Wci_B'/Subsystem/Subsystem1 ==
  1 : Inport
  Demux : Demux  Outputs=3
  skew : MATLAB Function  TreatAsAtomicUnit=on
  "skew " : Outport
  wires:
  1/1 -> Demux/1
  Demux/3 -> skew/3(a_3)
  Demux/2 -> skew/2(a_2)
  Demux/1 -> skew/1(a_1)
  skew/1(skew) -> "skew "/1

== system model_fully_coupled/r_double_dot_BN/c_double_dot/r_dprime_Wci_B/r_Wci_B'/Subsystem/Subsystem2 ==
  1 : Inport
  Demux : Demux  Outputs=3
  skew : MATLAB Function  TreatAsAtomicUnit=on
  "skew " : Outport
  wires:
  1/1 -> Demux/1
  Demux/3 -> skew/3(a_3)
  Demux/2 -> skew/2(a_2)
  Demux/1 -> skew/1(a_1)
  skew/1(skew) -> "skew "/1

== system model_fully_coupled/r_double_dot_BN/c_double_dot/r_dprime_Wci_B/r_Wci_B'/Subsystem/r"_Wc1_B ==
  OMEGA_1 : Inport
  g_s_1 : Inport  Port=2
  Matrix Multiply : Product  Multiplication=Matrix(*)
  Product : Product
  Subsystem1 : Subsystem
  Out1 : Outport
  tag scope: r_dprime_Wc1_B=global
  wires:
  Matrix Multiply/1 -> [r_dprime_Wc1_B], Out1/1
  [r_prime_Wc1_B] -> Matrix Multiply/2
  Subsystem1/1("skew ") -> Matrix Multiply/1
  Product/1 -> Subsystem1/1(1)
  OMEGA_1/1 -> Product/1
  g_s_1/1 -> Product/2

== system model_fully_coupled/r_double_dot_BN/c_double_dot/r_dprime_Wci_B/r_Wci_B'/Subsystem/r'_Wc1_B ==
  d_1 : Inport
  Product : Product
  1 : Outport
  wires:
  d_1/1 -> Product/1
  Product/1 -> 1/1
  [w_2_1_prime] -> Product/2

== system model_fully_coupled/r_double_dot_BN/c_double_dot/r_dprime_Wci_B/r_Wci_B'/Subsystem/r_Wc1_B ==
  r_W1_B : Inport
  d_1 : Inport  Port=2
  w_2_1 : Inport  Port=3
  Add : Sum
  Product : Product
  1 : Outport
  wires:
  r_W1_B/1 -> Add/1
  Product/1 -> Add/2
  d_1/1 -> Product/1
  w_2_1/1 -> Product/2
  Add/1 -> 1/1

== system model_fully_coupled/r_double_dot_BN/c_double_dot/r_dprime_Wci_B/r_Wci_B'/Subsystem1/Subsystem1 ==
  1 : Inport
  Demux : Demux  Outputs=3
  skew : MATLAB Function  TreatAsAtomicUnit=on
  "skew " : Outport
  wires:
  1/1 -> Demux/1
  Demux/3 -> skew/3(a_3)
  Demux/2 -> skew/2(a_2)
  Demux/1 -> skew/1(a_1)
  skew/1(skew) -> "skew "/1

== system model_fully_coupled/r_double_dot_BN/c_double_dot/r_dprime_Wci_B/r_Wci_B'/Subsystem1/Subsystem2 ==
  1 : Inport
  Demux : Demux  Outputs=3
  skew : MATLAB Function  TreatAsAtomicUnit=on
  "skew " : Outport
  wires:
  1/1 -> Demux/1
  Demux/3 -> skew/3(a_3)
  Demux/2 -> skew/2(a_2)
  Demux/1 -> skew/1(a_1)
  skew/1(skew) -> "skew "/1

== system model_fully_coupled/r_double_dot_BN/c_double_dot/r_dprime_Wci_B/r_Wci_B'/Subsystem1/r"_Wc2_B ==
  OMEGA_2 : Inport
  g_s_2 : Inport  Port=2
  Matrix Multiply : Product  Multiplication=Matrix(*)
  Product : Product
  Subsystem1 : Subsystem
  Out1 : Outport
  tag scope: r_dprime_Wc2_B=global
  wires:
  Matrix Multiply/1 -> [r_dprime_Wc2_B], Out1/1
  [r_prime_Wc2_B] -> Matrix Multiply/2
  Subsystem1/1("skew ") -> Matrix Multiply/1
  Product/1 -> Subsystem1/1(1)
  g_s_2/1 -> Product/2
  OMEGA_2/1 -> Product/1

== system model_fully_coupled/r_double_dot_BN/c_double_dot/r_dprime_Wci_B/r_Wci_B'/Subsystem1/r'_Wc2_B ==
  d_2 : Inport
  Product2 : Product
  1 : Outport
  wires:
  Product2/1 -> 1/1
  d_2/1 -> Product2/1
  [w_2_2_prime] -> Product2/2

== system model_fully_coupled/r_double_dot_BN/c_double_dot/r_dprime_Wci_B/r_Wci_B'/Subsystem1/r_Wc2_B ==
  r_W2_B : Inport
  d_2 : Inport  Port=2
  w_2_2 : Inport  Port=3
  Add1 : Sum
  Product1 : Product
  1 : Outport
  wires:
  r_W2_B/1 -> Add1/1
  w_2_2/1 -> Product1/2
  d_2/1 -> Product1/1
  Product1/1 -> Add1/2
  Add1/1 -> 1/1

== system model_fully_coupled/r_double_dot_BN/c_double_dot/r_dprime_Wci_B/r_Wci_B'/Subsystem2/Subsystem1 ==
  1 : Inport
  Demux : Demux  Outputs=3
  skew : MATLAB Function  TreatAsAtomicUnit=on
  "skew " : Outport
  wires:
  1/1 -> Demux/1
  Demux/3 -> skew/3(a_3)
  Demux/2 -> skew/2(a_2)
  Demux/1 -> skew/1(a_1)
  skew/1(skew) -> "skew "/1

== system model_fully_coupled/r_double_dot_BN/c_double_dot/r_dprime_Wci_B/r_Wci_B'/Subsystem2/Subsystem2 ==
  1 : Inport
  Demux : Demux  Outputs=3
  skew : MATLAB Function  TreatAsAtomicUnit=on
  "skew " : Outport
  wires:
  1/1 -> Demux/1
  Demux/3 -> skew/3(a_3)
  Demux/2 -> skew/2(a_2)
  Demux/1 -> skew/1(a_1)
  skew/1(skew) -> "skew "/1

== system model_fully_coupled/r_double_dot_BN/c_double_dot/r_dprime_Wci_B/r_Wci_B'/Subsystem2/r"_Wc3_B ==
  OMEGA_3 : Inport
  g_s_3 : Inport  Port=2
  Matrix Multiply : Product  Multiplication=Matrix(*)
  Product : Product
  Subsystem1 : Subsystem
  Out1 : Outport
  tag scope: r_dprime_Wc3_B=global
  wires:
  Matrix Multiply/1 -> [r_dprime_Wc3_B], Out1/1
  [r_prime_Wc3_B] -> Matrix Multiply/2
  Product/1 -> Subsystem1/1(1)
  Subsystem1/1("skew ") -> Matrix Multiply/1
  g_s_3/1 -> Product/2
  OMEGA_3/1 -> Product/1
